simulink model "sim"  (R2017b)
settings: Solver=VariableStepAuto  StartTime=0.0  StopTime=10.0  RelTol=1e-3
undefined symbols (not defined in the file or in its folder): B, g, J, m
libraries: fuzblock x1
settings Model: Creator=Estudiantes  LastModifiedBy=Estudiantes

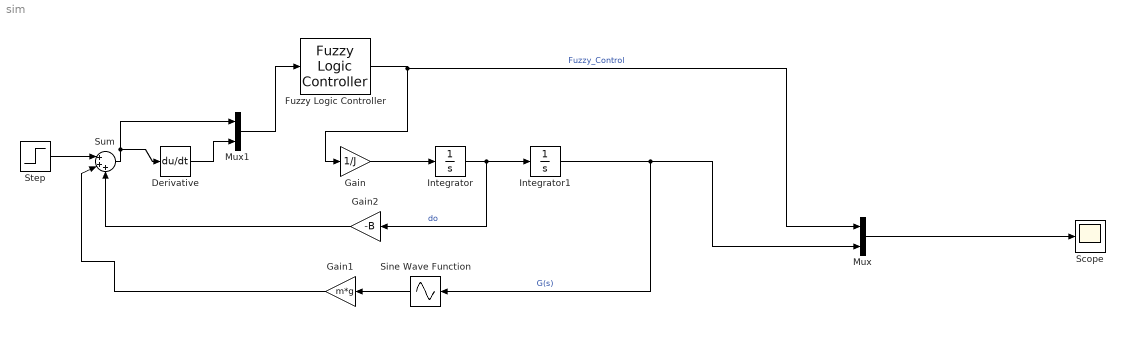
== system sim ==
  Derivative : Derivative
  Fuzzy Logic Controller : fuzblock/Fuzzy Logic  Controller  FIS=pendf  OutputSampleNumber=101  DataType=double  FuzzifiedInputs=off  RuleFiringStrengths=off  RuleOutputs=off  AggregatedOutputs=off  SimulateUsing=Interpreted execution
  Gain : Gain  Gain=1/J
  Gain1 : Gain  Gain=m*g
  Gain2 : Gain  Gain=-B
  Integrator : Integrator
  Integrator1 : Integrator
  Mux : Mux  Inputs=2
  Mux1 : Mux  Inputs=2
  Scope : Scope
  Sine Wave Function : Sin  TimeSource=Use external signal  SampleTime=0
  Step : Step  SampleTime=0
  Sum : Sum  Inputs=|+++
  wires:
  Gain/1 -> Integrator/1
  Integrator/1 -> Gain2/1, Integrator1/1  "do"
  Gain1/1 -> Sum/2
  Sine Wave Function/1 -> Gain1/1
  Integrator1/1 -> Mux/2, Sine Wave Function/1  "G(s)"
  Gain2/1 -> Sum/3
  Mux/1 -> Scope/1
  Step/1 -> Sum/1
  Fuzzy Logic Controller/1 -> Mux/1, Gain/1  "Fuzzy_Control"
  Mux1/1 -> Fuzzy Logic Controller/1
  Sum/1 -> Derivative/1, Mux1/1
  Derivative/1 -> Mux1/2
